simulink model "InC_Dynamic"  (R2024b)
settings: Solver=VariableStepAuto  StartTime=0.0  StopTime=23  RelTol=1e-3
undefined symbols (not defined in the file): Irradiance
libraries: spsSeriesRLCBranchLib x6, spsCurrentMeasurementLib x2, spsVoltageMeasurementLib x2, spsPVArrayLib x1, spsPWMGeneratorDCDCLib x1, spsDiodeLib x1, spsIGBTDiodeLib x1, spspowerguiLib x1
settings Model: Creator=Venkatesh  LastModifiedBy=aniru
settings DebuggingCC: UnconnectedInputMsg=warning  UnconnectedOutputMsg=warning  UnconnectedLineMsg=warning
settings ModelReferenceCC: EnableRefExpFcnMdlSchedulingChecks=on
settings RTWCC: GPUComputeCapability=3.5  DLArmComputeVersion=19.05

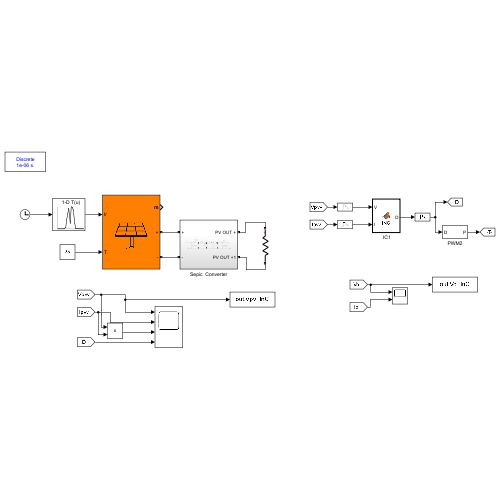
[thumbnail: Simulink's stored preview of the top-level diagram]
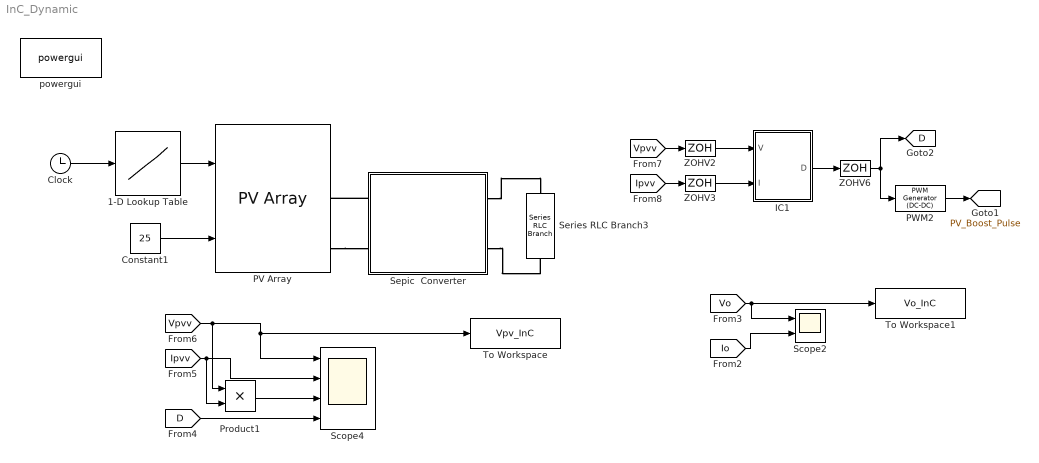
== system InC_Dynamic ==
  " IC1" : MATLAB Function  TreatAsAtomicUnit=on
  1-D Lookup Table : Lookup_n-D  NumberOfTableDimensions=1  BreakpointsForDimension1=0:23  Table=Irradiance  InternalRulePriority=Speed  RndMeth=Simplest
  Clock : Clock
  Constant1 : Constant  Value=25
  PV Array : spsPVArrayLib/PV Array  Npar=1  Nser=4  PlotType=array @ 1000 W/m2 & specified temperatures  S_vec="[ 1000  500  100 ]"  Temp_C_vec="[ 45 25  ]"  ModuleName=User-defined  PlotWhenSelected=off  Pm=301.928  Ncell=72  Voc=44.5  Isc=8.5  Vm=37.6  Im=8.03  beta_Voc_pc=-0.3631  alpha_Isc_pc=0.084299  beta_Voc=-0.16158  alpha_Isc=0.0071654  IL=8.5518  I0=3.3263e-10  nI=1.0044  Rsh=258.384  Rs=0.15735  RobustModel=off  RobustCellTemperature=313.3991  BAL=off  Tc=1e-6  Tfilter=5e-5
  PWM2 : spsPWMGeneratorDCDCLib/PWM Generator (DC-DC)  Fsw=10000  Ts=1e-6
  Product1 : Product
  Scope2 : Scope  NumInputPorts=2
  Scope4 : Scope  NumInputPorts=4
  Sepic  Converter : Subsystem
  Series RLC Branch3 : spsSeriesRLCBranchLib/Series RLC Branch  LConnTagsString=__new0  RConnTagsString=__new0  BranchType=R  Resistance=7  Inductance=3e-3  SetiL0=off  InitialCurrent=0  Capacitance=1e-6  Setx0=off  InitialVoltage=0  Measurements=None
  To Workspace : ToWorkspace  VariableName=Vpv_InC  SampleTime=-1
  To Workspace1 : ToWorkspace  VariableName=Vo_InC  SampleTime=-1
  ZOHV2 : ZeroOrderHold  SampleTime=0.02
  ZOHV3 : ZeroOrderHold  SampleTime=0.02
  ZOHV6 : ZeroOrderHold  SampleTime=0.02
  powergui : spspowerguiLib/powergui  Priority=1  SimulationMode=Discrete  SampleTime=1e-6  frequency=60  Iterations=50  frequencyindice=0  Pbase=100e6  ErrMax=1e-4  UnitsV=kV  UnitsW=MW  buscounter=0  FunctionMessages=off  echomessages=off  EnableUseOfTLC=off  CurrentSourceSwitches=off  DisableSnubberDevices=off  DisableRonSwitches=off  DisableVfSwitches=off  DisplayEquations=off  AutomaticDiscreteSolvers=off  SolverType=Tustin/Backward Euler (TBE)  Interpol=off  ExternalGateDelay=off  methode=off  Ts=100  x0status=blocks  SPID=on  SwTol=0  HookPort=off  NonlinearTolerance=1e-4  nMaxIteration=100  ContinueOnMaxIteration=off  RestoreLinks=warning  ResistiveCurrentMeasurement=off  Frange=[0:2:500]  Ylog=off  Xlog=on  ShowGrid=off  save=off  variable=ZData  structure=0  ZoomFFT=off  StartTime=0.0  cycles=1  DisplayStyle=1  fundamental=60  FreqAxis=off  MaxFrequency=1000  frequencyindicesteady=1  RmsSteady=1  display=off
  tag scope: D=global, PV_Boost_Pulse=global
  wires:
  [Vpvv] -> Product1/1, To Workspace/1, Scope4/1
  [D] -> Scope4/4
  ZOHV6/1 -> [D], PWM2/1
  ZOHV3/1 -> " IC1"/2(I)
  [Ipvv] -> ZOHV3/1
  " IC1"/1(D) -> ZOHV6/1
  [Io] -> Scope2/2
  [Vpvv] -> ZOHV2/1
  ZOHV2/1 -> " IC1"/1(V)
  PWM2/1 -> [PV_Boost_Pulse]
  Product1/1 -> Scope4/3
  [Vo] -> To Workspace1/1, Scope2/1
  Constant1/1 -> PV Array/2
  [Ipvv] -> Product1/2, Scope4/2
  1-D Lookup Table/1 -> PV Array/1
  Clock/1 -> 1-D Lookup Table/1
  connections:
  PV Array/RConn2 -- Sepic  Converter/LConn2
  Sepic  Converter/LConn1 -- PV Array/RConn1
  Sepic  Converter/RConn2 -- Series RLC Branch3/RConn1
  Sepic  Converter/RConn1 -- Series RLC Branch3/LConn1

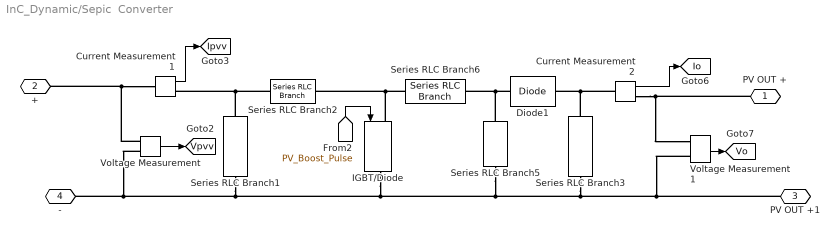
== system InC_Dynamic/Sepic  Converter ==
  Current Measurement1 : spsCurrentMeasurementLib/Current Measurement  PhasorSimulation=off  OutputType=Complex  PSBequivalent=0
  Current Measurement2 : spsCurrentMeasurementLib/Current Measurement  PhasorSimulation=off  OutputType=Complex  PSBequivalent=0
  Diode1 : spsDiodeLib/Diode  Ron=0.001  Lon=0  Vf=0.8  IC=0  UseSnubber=off  Rs=inf  Cs=250e-9  Measurements=off
  IGBT/Diode : spsIGBTDiodeLib/IGBT//Diode  Ron=1e-3  Rs=1e5  Cs=inf  Measurements=off
  Series RLC Branch1 : spsSeriesRLCBranchLib/Series RLC Branch  LConnTagsString=__new0  RConnTagsString=__new0  BranchType=C  Resistance=0.001  Inductance=3e-3  SetiL0=off  InitialCurrent=0  Capacitance=47e-6  Setx0=off  InitialVoltage=150  Measurements=None
  Series RLC Branch2 : spsSeriesRLCBranchLib/Series RLC Branch  LConnTagsString=__new0  RConnTagsString=__new0  BranchType=RL  Resistance=1  Inductance=3.3e-3  SetiL0=off  InitialCurrent=0  Capacitance=1e-6  Setx0=off  InitialVoltage=0  Measurements=None
  Series RLC Branch3 : spsSeriesRLCBranchLib/Series RLC Branch  LConnTagsString=__new0  RConnTagsString=__new0  BranchType=RC  Resistance=0.001  Inductance=3e-3  SetiL0=off  InitialCurrent=0  Capacitance=220e-6  Setx0=off  InitialVoltage=150  Measurements=None
  Series RLC Branch5 : spsSeriesRLCBranchLib/Series RLC Branch  LConnTagsString=__new0  RConnTagsString=__new0  BranchType=RL  Resistance=1  Inductance=3.3e-3  SetiL0=off  InitialCurrent=0  Capacitance=1e-6  Setx0=off  InitialVoltage=0  Measurements=None
  Series RLC Branch6 : spsSeriesRLCBranchLib/Series RLC Branch  LConnTagsString=__new0  RConnTagsString=__new0  BranchType=RC  Resistance=1  Inductance=3e-3  SetiL0=off  InitialCurrent=0  Capacitance=47e-6  Setx0=off  InitialVoltage=150  Measurements=None
  Voltage Measurement : spsVoltageMeasurementLib/Voltage Measurement  PhasorSimulation=off  OutputType=Complex  PSBequivalent=0
  Voltage Measurement1 : spsVoltageMeasurementLib/Voltage Measurement  PhasorSimulation=off  OutputType=Complex  PSBequivalent=0
  PV OUT + : PMIOPort  Side=Right
  + : PMIOPort  Port=2  Side=Left
  PV OUT +1 : PMIOPort  Port=3  Side=Right
  - : PMIOPort  Port=4  Side=Left
  tag scope: Io=global, Ipvv=global, Vo=global, Vpvv=global
  wires:
  Current Measurement1/1 -> [Ipvv]
  Current Measurement2/1 -> [Io]
  [PV_Boost_Pulse] -> IGBT/Diode/1
  Voltage Measurement/1 -> [Vpvv]
  Voltage Measurement1/1 -> [Vo]
  connections:
  Voltage Measurement/LConn1 -- Current Measurement1/LConn1 -- +/RConn1
  PV OUT +1/RConn1 -- Voltage Measurement1/LConn2 -- Series RLC Branch3/RConn1 -- Series RLC Branch5/RConn1 -- IGBT/Diode/RConn1 -- Series RLC Branch1/RConn1 -- Voltage Measurement/LConn2 -- -/RConn1
  PV OUT +/RConn1 -- Current Measurement2/RConn1 -- Voltage Measurement1/LConn1
  Series RLC Branch1/LConn1 -- Series RLC Branch2/LConn1 -- Current Measurement1/RConn1
  IGBT/Diode/LConn1 -- Series RLC Branch6/RConn1 -- Series RLC Branch2/RConn1
  Series RLC Branch5/LConn1 -- Series RLC Branch6/LConn1 -- Diode1/LConn1
  Current Measurement2/LConn1 -- Series RLC Branch3/LConn1 -- Diode1/RConn1

== matlab function InC_Dynamic/ IC1 ==
  data: V input; I input; D output
% f=10000 hz 
function D  = INC(V, I)
 
 
Dinit = 0.5;  %Initial value for D output
Dmax = 0.8;   %Maximum value for D
Dmin = 0.1;   %Minimum value for D
deltaD = 0.01; %Increment value used to increase/decrease the duty cycle D
 
  
persistent Vold Dold Iold;
 
dataType = 'double';
 
if isempty(Vold)
    Vold=0;
    Iold=0;
    Dold=Dinit;
end
dV= V - Vold;
dI= I - Iold;
 
    if dV == 0
        if dI == 0
            D=Dold;
        else
           if dI > 0
            D = Dold - deltaD;
           else 
            D = Dold + deltaD;
           end
        end
    else
        if (dI/dV) == -(I/V)
            D=Dold;
        else
            if (dI/dV) > -(I/V)
           D=Dold - deltaD;
            else
           D=Dold + deltaD;  
            end 
        end
    end    
 
if D >= Dmax || D<= Dmin
    D=Dold;
end
 
Dold=D;
Vold=V;
Iold=I;
